simulink model "TP2"  (R2016b)
settings: Solver=VariableStepAuto  StartTime=0.0  StopTime=500  RelTol=1e-3
undefined symbols (not defined in the file or in its folder): Constant1
libraries: dspinverses x1
settings Model: Creator=Nahkriin  LastModifiedBy=Nahkriin

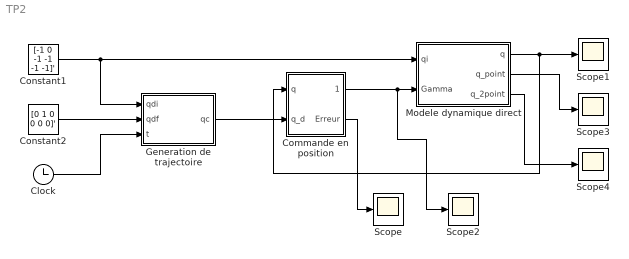
== system TP2 ==
  Clock : Clock
  Commande en position : Subsystem
  Constant1 : Constant  Value=[-1 0 -1 -1 -1 -1]'  VectorParams1D=off
  Constant2 : Constant  Value=[0 1 0 0 0 0]'  VectorParams1D=off
  Generation de trajectoire : MATLAB Function  TreatAsAtomicUnit=on
  Modele dynamique direct : Subsystem
  Scope{,1..4} (5 alike) : Scope
  wires:
  Constant1/1 -> Generation de trajectoire/1(qdi), Modele dynamique direct/1(qi)
  Constant2/1 -> Generation de trajectoire/2(qdf)
  Clock/1 -> Generation de trajectoire/3(t)
  Modele dynamique direct/1("q ") -> Commande en position/1(q), Scope1/1
  Generation de trajectoire/1(qc) -> Commande en position/2("q_d ")
  Commande en position/1("Gamma ") -> Scope2/1, Modele dynamique direct/2(Gamma)
  Commande en position/2("Erreur ") -> Scope/1
  Modele dynamique direct/2("q_point ") -> Scope3/1
  Modele dynamique direct/3(q_2point) -> Scope4/1

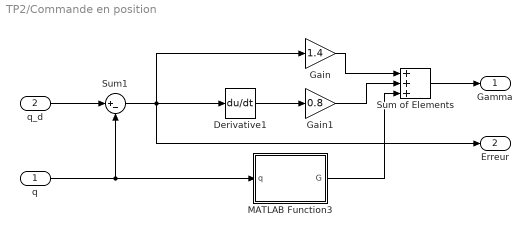
== system TP2/Commande en position ==
  q : Inport
  "q_d " : Inport  Port=2
  Derivative1 : Derivative
  Gain : Gain  Gain=1.4
  Gain1 : Gain  Gain=0.8
  MATLAB Function3 : MATLAB Function  TreatAsAtomicUnit=on
  Sum of Elements : Sum  Inputs=+++
  Sum1 : Sum  Inputs=|+-
  "Gamma " : Outport
  "Erreur " : Outport  Port=2
  wires:
  Sum of Elements/1 -> "Gamma "/1
  q/1 -> Sum1/2, MATLAB Function3/1(q)
  Derivative1/1 -> Gain1/1
  "q_d "/1 -> Sum1/1
  Gain/1 -> Sum of Elements/1
  Gain1/1 -> Sum of Elements/2
  MATLAB Function3/1(G) -> Sum of Elements/3
  Sum1/1 -> "Erreur "/1, Gain/1, Derivative1/1

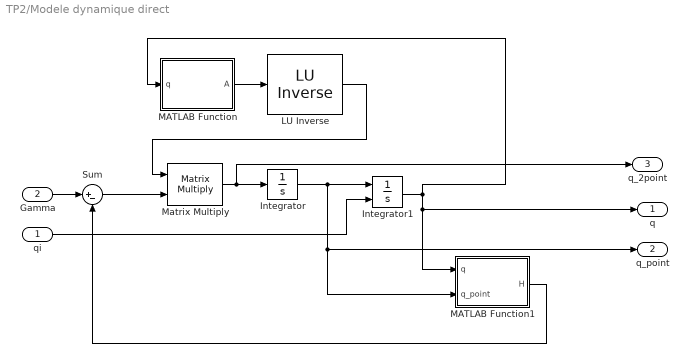
== system TP2/Modele dynamique direct ==
  qi : Inport
  Gamma : Inport  Port=2
  " LU Inverse" : dspinverses/ LU Inverse
  Integrator : Integrator  InitialCondition=[0 0 0 0 0 0]'
  Integrator1 : Integrator  InitialConditionSource=external  InitialCondition=Constant1
  MATLAB Function : MATLAB Function  TreatAsAtomicUnit=on
  MATLAB Function1 : MATLAB Function  TreatAsAtomicUnit=on
  Matrix Multiply : Product  Multiplication=Matrix(*)
  Sum : Sum  Inputs=|+-
  "q " : Outport
  "q_point " : Outport  Port=2
  q_2point : Outport  Port=3
  wires:
  qi/1 -> Integrator1/2
  " LU Inverse"/1 -> Matrix Multiply/1
  Sum/1 -> Matrix Multiply/2
  Matrix Multiply/1 -> q_2point/1, Integrator/1
  Integrator1/1 -> MATLAB Function/1(q), MATLAB Function1/1(q), "q "/1
  Gamma/1 -> Sum/1
  MATLAB Function/1(A) -> " LU Inverse"/1
  Integrator/1 -> "q_point "/1, MATLAB Function1/2(q_point), Integrator1/1
  MATLAB Function1/1(H) -> Sum/2

== matlab function TP2/Modele dynamique direct/MATLAB Function1 ==
  data: q input; H output; q_point input
function H  = CalculMatriceH(q,q_point)
    H = CalculCoupleCoriolisCentrifuge(q,q_point) + CalculCoupleGravite(q) + CalculCoupleFrottement(q_point);
end

== matlab function TP2/Modele dynamique direct/MATLAB Function ==
  data: A output; q input
function A = CalculMatriceInertie(q)

    %Parametres geometriques du robot - Convention DHM
    d3 = 0.7;
    r1 = 0.5;
    r4 = 0.2;

    alpha = [0 pi/2 0 pi/2 -pi/2 pi/2];
    d = [0 0 d3 0 0 0];
    r = [r1 0 0 r4 0 0];

    %Parametres inertiels du robot

    m = [15 10 1 7 1 0.5];
    OG = [0 0 -0.25;0.35 0 0;0 -0.1 0; 0 0 0;0 0 0;0 0 0];

    I = [[0.8 0 0.05;0 0.8 0;0.05 0 0.1];
        [0.1 0 0.1;0 1.5 0;0.1 0 1.5];
        [0.05 0 0;0 0.01 0;0 0 0.05];
        [0.5 0 0;0 0.5 0;0 0 0.5];
        [0.01 0 0;0 0.01 0;0 0 0.01];
        [0.01 0 0;0 0.01 0;0 0 0.01]];

    %Paramètres inertiels des rotors

    Rred = [100 100 100 70 70 70];
    Jm = ones(size(Rred))*10^(-5);

    theta = [q(1) q(2) q(3)+pi/2 q(4) q(5) q(6)].';
    g_0i = eye(4);

    Ig = zeros(3*size(q,1),3);
    for i = 1:length(m)
        Huy = [OG(i,2)^2+OG(i,3)^2 -OG(i,1)*OG(i,2) -OG(i,1)*OG(i,3);
                -OG(i,1)*OG(i,2) OG(i,1)^2+OG(i,3)^2 -OG(i,2)*OG(i,3);
                -OG(i,1)*OG(i,3) -OG(i,2)*OG(i,3) OG(i,1)^2+OG(i,2)^2];
        
        g_elem = CalculTransformationElem(alpha(i),d(i),theta(i),r(i));
        g_0i = g_0i*g_elem;
        ROi = g_0i(1:3,1:3);

        Ig(3*(i-1)+1:3*i,:) = ROi*(I(3*(i-1)+1:3*i,:)-m(i).*Huy)*ROi.';        
    end

    theta = [q(1) q(2) q(3)+pi/2 q(4) q(5) q(6)];  
    
    [OJv_Gi, OJ_wi] = CalculMatriceJacobienneGi(alpha, d, theta, r, OG(:,1), OG(:,2), OG(:,3));

    A = zeros(size(theta,2),size(theta,2));
    for i=1:size(theta,2) 
        A = A + OJv_Gi(:,:,i).'*OJv_Gi(:,:,i)*m(i)+ OJ_wi(:,:,i).'*Ig(3*(i-1)+1:3*i,:)*OJ_wi(:,:,i);
    end
   
    A = A + diag(Rred.^2.*Jm);

end

== matlab function TP2/Generation de trajectoire ==
  data: qdi input; qc output; qdf input; t input
function qc  = GeneTraj(qdi,qdf,t)
    tf = 500;
    D = qdf - qdi;
    
    r = 10*(t/tf)^3 - 15*(t/tf)^4 + 6*(t/tf)^5;
    
    qc = qdi + D*r;
end

== matlab function TP2/Commande en position/MATLAB Function3 ==
  data: q input; G output
function G  = CalculCoupleGravite(q)
    g = [0 0 -9.81].';  
    
    %Global variables => Doesn't work well with simulink
    %global alpha d r OG m;
    
    %Parametres geometriques du robot - Convention DHM
    d3 = 0.7;
    r1 = 0.5;
    r4 = 0.2;

    alpha = [0 pi/2 0 pi/2 -pi/2 pi/2];
    d = [0 0 d3 0 0 0];
    r = [r1 0 0 r4 0 0];

    %Parametres inertiels du robot

    m = [15 10 1 7 1 0.5];
    OG = [0 0 -0.25;0.35 0 0;0 -0.1 0; 0 0 0;0 0 0;0 0 0];
    
    theta = [q(1) q(2) q(3)+pi/2 q(4) q(5) q(6)].';
    
    [OJv_Gi, ~] = CalculMatriceJacobienneGi(alpha, d, theta, r, OG(:,1),OG(:,2),OG(:,3));
    
    G = zeros(size(theta));
    
    for i=1:size(theta,1)
       G = G + OJv_Gi(:,:,i).'*m(i)*g;
    end
    
    G = -G;
end
